simulink model "distillmpcbasic"  (Simulink 6.6)
settings: Solver=ode45  StartTime=0.0  StopTime=100.0  RelTol=1e-3
values from neighbouring files (symbols this model uses):
  alpha = 2.993    [distilldata.mat]
  F = block.DialogPrm(1).Data    [mympccontroller.m]    (also in run_lab3_5_1.m = sysd.A; run_lab3_5_2.m = sysd.A; run_lab3_5_3.m = sysd.A)
  F0 = 1    [distilldata.mat]
  G = block.DialogPrm(2).Data    [mympccontroller.m]    (also in run_lab3_5_1.m = sysd.B; run_lab3_5_2.m = sysd.B; run_lab3_5_3.m = sysd.B)
  L0 = 2    [distilldata.mat]
  M = 5    [distilldata.mat]    (also in mympccontroller.m = block.DialogPrm(3).Data; upg_10_1.m = eye(m); upg_10_2.m = eye(m))
  M0B = 10    [distilldata.mat]
  M0D = 10    [distilldata.mat]
  Mz = [1 0 0 0 0 0 0 0 0 0 0 0 ... (16 elements, 2x8)]    [distilldata.mat]    (also in run_lab3_5_3.m = [Mz, zeros(size(Mz,1),1); zeros(1,size(Mz,2)), 1])
  N = block.DialogPrm(4).Data    [mympccontroller.m]    (also in results_51.mat = 20; run_lab3_5_1.m = 20; run_lab3_5_2.m = 70; run_lab3_5_3.m = 70)
  Q1 = block.DialogPrm(5).Data    [mympccontroller.m]    (also in run_lab3_5_1.m = eye(size(Mz,1)); run_lab3_5_2.m = diag([110, 200]); run_lab3_5_3.m = diag([110, 200, q_z3]); upg_10_1.m = 10*eye(m))
  Q2 = block.DialogPrm(6).Data    [mympccontroller.m]    (also in run_lab3_5_1.m = 1e-2*eye(size(G,2)); run_lab3_5_2.m = 6e-4*eye(m); run_lab3_5_3.m = diag([1,1 1000]); upg_10_1.m = 0.1)
  Ts = block.DialogPrm(8).Data    [mympccontroller.m]    (also in results_51.mat = 1; run_lab3_5_1.m = 1; run_lab3_5_2.m = 1; run_lab3_5_3.m = 1)
  ubounds = block.DialogPrm(7).Data    [mympccontroller.m]    (also in results_51.mat = [-2.5  2.5; -2  3]; run_lab3_5_1.m = [ -V0, 5 - V0; run_lab3_5_2.m = [ -V0, 5 - V0; run_lab3_5_3.m = [ -V0, 5 - V0)
  V0 = 2.5    [distilldata.mat]
  x0 = [0.9577452092 0.883354566 0.7467709401 0.5553784995 0.3912960402 0.2223240273 0.1042469935 0.04225479085]    [distilldata.mat]    (also in run_lab3_5_1.m = xdagger; run_lab3_5_2.m = xstar(:); run_lab3_5_3.m = xstar(:))
  xF0 = 0.5    [distilldata.mat]
  xstar = [0.9577452092 0.883354566 0.7467709401 0.5553784995 0.3912960402 0.2223240273 0.1042469935 0.04225479085]    [distilldata.mat]
settings Model: Creator=maren  LastModifiedBy=maren  ExtModeAutoUpdateStatusClock=off

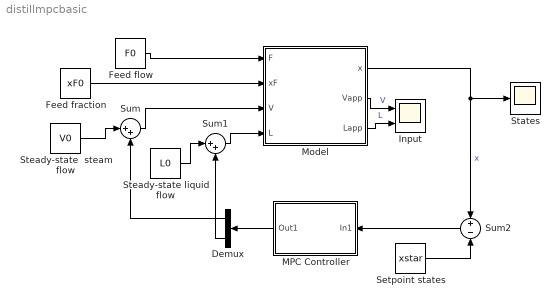
== system distillmpcbasic ==
  Demux : Demux  Orientation=left  Outputs=2
  Feed flow : Constant  Value=F0
  Feed fraction : Constant  Value=xF0
  Input : Scope  NumInputPorts=2
      settings: TimeRange=100  YMin=2.5~2  YMax=5~2.125  SaveName=U
  MPC Controller : Subsystem  Orientation=left  mask{F=F, G=G, M=Mz, N=N, Q1=Q1, Q2=Q2, ubounds=ubounds, Ts=Ts, ufname='solvempcproblem'}
      mask prompts: ubounds "Input bounds [u1min u1max;u2min u2max;...]"; ufname "Output function (Ex: 'myfun1')"
      mask Display:
      | port_label('input',1,'x')
      | port_label('output',1,'u')
  Model : Subsystem
  Setpoint states : Constant  Value=xstar
  States : Scope
      settings: TimeRange=100  YMin=0  YMax=1  SaveName=X
  Steady-state liquid flow : Constant  Value=L0
  Steady-state  steam flow : Constant  Value=V0
  Sum : Sum  Inputs=|++  SaturateOnIntegerOverflow=on
  Sum1 : Sum  Inputs=|++  SaturateOnIntegerOverflow=on
  Sum2 : Sum  Orientation=left  Inputs=+-  SaturateOnIntegerOverflow=on
  wires:
  Feed flow/1 -> Model/1(F)
  Feed fraction/1 -> Model/2(xF)
  Steady-state  steam flow/1 -> Sum/1
  Sum/1 -> Model/3(V)
  Demux/1 -> Sum/2
  Steady-state liquid flow/1 -> Sum1/1
  Demux/2 -> Sum1/2
  Sum1/1 -> Model/4(L)
  Model/1(x) -> States/1, Sum2/1  "x"
  Setpoint states/1 -> Sum2/2
  Model/2(Vapp) -> Input/1  "V"
  Model/3(Lapp) -> Input/2  "L"
  MPC Controller/1(Out1) -> Demux/1
  Sum2/1 -> MPC Controller/1(In1)

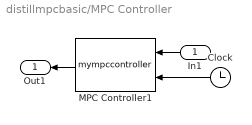
== system distillmpcbasic/MPC Controller ==
  In1 : Inport  Orientation=left
  Clock : Clock
      settings: Decimation=10
  MPC Controller1 : M-S-Function  Orientation=left  FunctionName=mympccontroller  Parameters=F,G,M,N,Q1,Q2,ubounds,Ts,ufname  mask{F=F, G=G, M=M, N=N, Q1=Q1, Q2=Q2, ubounds=ubounds, Ts=Ts, ufname=ufname}
      mask prompts: ubounds "ubounds [u1min u1max;u2min u2max;...]"; ufname "Output function (Ex: 'myfun1')"
      mask Display:
      | port_label('input',1,'x')
      | port_label('input',2,'t')
      | port_label('output',1,'u')
  Out1 : Outport  Orientation=left
  wires:
  Clock/1 -> MPC Controller1/2
  In1/1 -> MPC Controller1/1
  MPC Controller1/1 -> Out1/1

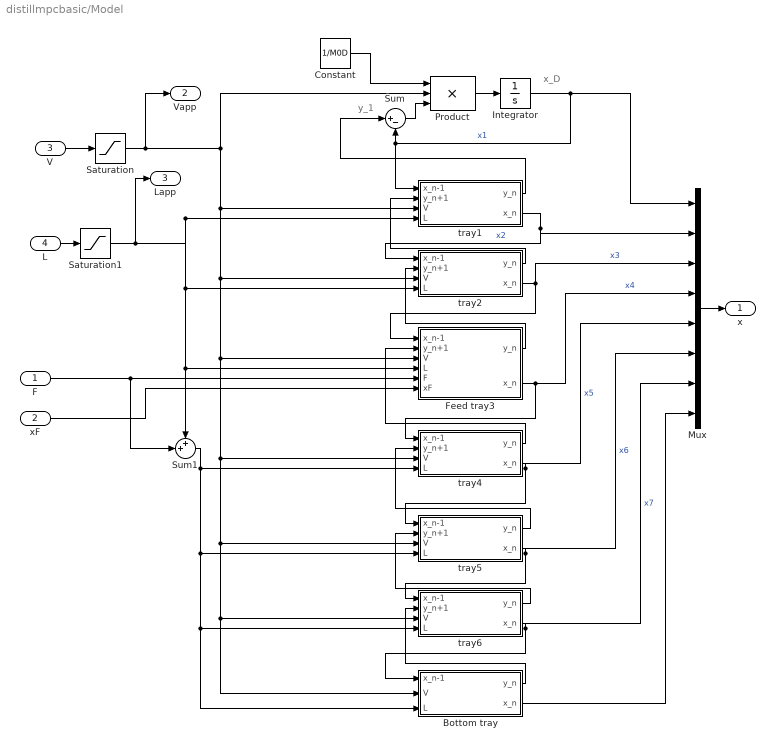
== system distillmpcbasic/Model ==
  note: y_1
  note: x_D
  F : Inport
  xF : Inport  Port=2
  V : Inport  Port=3
  L : Inport  Port=4
  Bottom tray : Subsystem
  Constant : Constant  Value=1/M0D
  Feed tray3 : Subsystem
  Integrator : Integrator  InitialCondition=x0(1)
  Mux : Mux  Inputs=8
  Product : Product  Inputs=3  SaturateOnIntegerOverflow=on
  Saturation : Saturate  UpperLimit=5  LowerLimit=0
  Saturation1 : Saturate  UpperLimit=5  LowerLimit=0
  Sum : Sum  Inputs=|+-  SaturateOnIntegerOverflow=on
  Sum1 : Sum  Inputs=++|  SaturateOnIntegerOverflow=on
  tray1 : Subsystem
  tray2 : Subsystem
  tray4 : Subsystem
  tray5 : Subsystem
  tray6 : Subsystem
  x : Outport
  Vapp : Outport  Port=2
  Lapp : Outport  Port=3
  wires:
  L/1 -> Saturation1/1
  V/1 -> Saturation/1
  Mux/1 -> x/1
  Bottom tray/2(x_n) -> Mux/8
  tray6/2(x_n) -> Mux/7, Bottom tray/1(x_n-1)  "x7"
  Bottom tray/1(y_n) -> tray6/2(y_n+1)
  Sum1/1 -> Bottom tray/3(L), tray6/4(L), tray5/4(L), tray4/4(L)
  tray5/2(x_n) -> Mux/6, tray6/1(x_n-1)  "x6"
  tray6/1(y_n) -> tray5/2(y_n+1)
  tray4/2(x_n) -> Mux/5, tray5/1(x_n-1)  "x5"
  tray5/1(y_n) -> tray4/2(y_n+1)
  Feed tray3/2(x_n) -> Mux/4, tray4/1(x_n-1)  "x4"
  tray4/1(y_n) -> Feed tray3/2(y_n+1)
  xF/1 -> Feed tray3/6(xF)
  F/1 -> Sum1/2, Feed tray3/5(F)
  tray2/2(x_n) -> Mux/3, Feed tray3/1(x_n-1)  "x3"
  Feed tray3/1(y_n) -> tray2/2(y_n+1)
  tray1/2(x_n) -> Mux/2, tray2/1(x_n-1)  "x2"
  tray2/1(y_n) -> tray1/2(y_n+1)
  tray1/1(y_n) -> Sum/1
  Saturation1/1 -> Lapp/1, Sum1/1, Feed tray3/4(L), tray2/4(L), tray1/4(L)
  Saturation/1 -> Vapp/1, Bottom tray/2(V), tray6/3(V), tray5/3(V), tray4/3(V), Feed tray3/3(V), tray2/3(V), tray1/3(V), Product/2
  Sum/1 -> Product/3
  Constant/1 -> Product/1
  Product/1 -> Integrator/1
  Integrator/1 -> Mux/1, tray1/1(x_n-1), Sum/2  "x1"

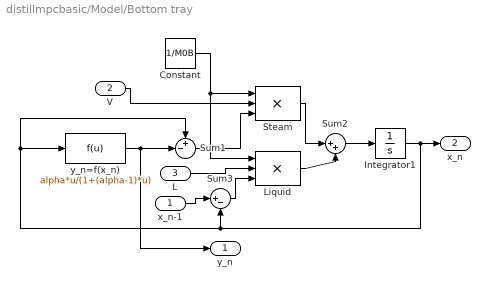
== system distillmpcbasic/Model/Bottom tray ==
  x_n-1 : Inport
  V : Inport  Port=2
  L : Inport  Port=3
  Constant : Constant  Value=1/M0B
  Integrator1 : Integrator  InitialCondition=x0(8)
  Liquid : Product  Inputs=3  SaturateOnIntegerOverflow=on
  Steam : Product  Inputs=3  SaturateOnIntegerOverflow=on
  Sum1 : Sum  Inputs=+-|  SaturateOnIntegerOverflow=on
  Sum2 : Sum  Inputs=|++  SaturateOnIntegerOverflow=on
  Sum3 : Sum  Inputs=|+-  SaturateOnIntegerOverflow=on
  y_n=f(x_n) : Fcn  Expr=alpha*u/(1+(alpha-1)*u)
  y_n : Outport
  x_n : Outport  Port=2
  wires:
  Sum1/1 -> Steam/3
  Constant/1 -> Steam/1, Liquid/1
  Integrator1/1 -> x_n/1, Sum1/1, y_n=f(x_n)/1, Sum3/2
  y_n=f(x_n)/1 -> y_n/1, Sum1/2
  V/1 -> Steam/2
  Liquid/1 -> Sum2/2
  Steam/1 -> Sum2/1
  Sum2/1 -> Integrator1/1
  L/1 -> Liquid/2
  x_n-1/1 -> Sum3/1
  Sum3/1 -> Liquid/3

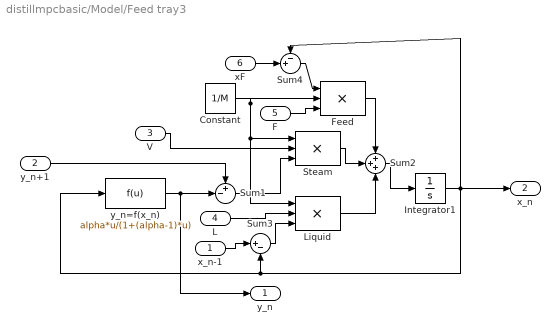
== system distillmpcbasic/Model/Feed tray3 ==
  x_n-1 : Inport
  y_n+1 : Inport  Port=2
  V : Inport  Port=3
  L : Inport  Port=4
  F : Inport  Port=5
  xF : Inport  Port=6
  Constant : Constant  Value=1/M
  Feed : Product  Inputs=3  SaturateOnIntegerOverflow=on
  Integrator1 : Integrator  InitialCondition=x0(4)
  Liquid : Product  Inputs=3  SaturateOnIntegerOverflow=on
  Steam : Product  Inputs=3  SaturateOnIntegerOverflow=on
  Sum1 : Sum  Inputs=+-|  SaturateOnIntegerOverflow=on
  Sum2 : Sum  Inputs=+++  SaturateOnIntegerOverflow=on
  Sum3 : Sum  Inputs=|+-  SaturateOnIntegerOverflow=on
  Sum4 : Sum  Inputs=-+|  SaturateOnIntegerOverflow=on
  y_n=f(x_n) : Fcn  Expr=alpha*u/(1+(alpha-1)*u)
  y_n : Outport
  x_n : Outport  Port=2
  wires:
  Feed/1 -> Sum2/1
  Sum4/1 -> Feed/1
  F/1 -> Feed/3
  xF/1 -> Sum4/2
  Steam/1 -> Sum2/2
  Liquid/1 -> Sum2/3
  Sum1/1 -> Steam/3
  Constant/1 -> Feed/2, Steam/1, Liquid/1
  Integrator1/1 -> Sum4/1, x_n/1, y_n=f(x_n)/1, Sum3/2
  y_n=f(x_n)/1 -> y_n/1, Sum1/2
  y_n+1/1 -> Sum1/1
  V/1 -> Steam/2
  Sum2/1 -> Integrator1/1
  L/1 -> Liquid/2
  x_n-1/1 -> Sum3/1
  Sum3/1 -> Liquid/3

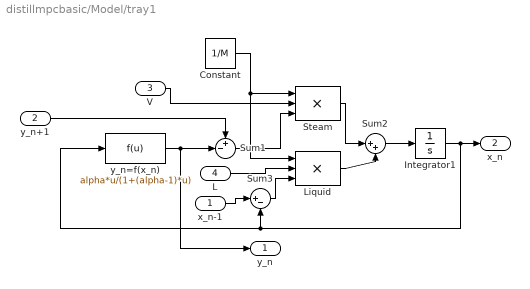
== system distillmpcbasic/Model/tray1 ==
  x_n-1 : Inport
  y_n+1 : Inport  Port=2
  V : Inport  Port=3
  L : Inport  Port=4
  Constant : Constant  Value=1/M
  Integrator1 : Integrator  InitialCondition=x0(2)
  Liquid : Product  Inputs=3  SaturateOnIntegerOverflow=on
  Steam : Product  Inputs=3  SaturateOnIntegerOverflow=on
  Sum1 : Sum  Inputs=+-|  SaturateOnIntegerOverflow=on
  Sum2 : Sum  Inputs=|++  SaturateOnIntegerOverflow=on
  Sum3 : Sum  Inputs=|+-  SaturateOnIntegerOverflow=on
  y_n=f(x_n) : Fcn  Expr=alpha*u/(1+(alpha-1)*u)
  y_n : Outport
  x_n : Outport  Port=2
  wires:
  Sum1/1 -> Steam/3
  Constant/1 -> Steam/1, Liquid/1
  Integrator1/1 -> x_n/1, y_n=f(x_n)/1, Sum3/2
  y_n=f(x_n)/1 -> y_n/1, Sum1/2
  y_n+1/1 -> Sum1/1
  V/1 -> Steam/2
  Liquid/1 -> Sum2/2
  Steam/1 -> Sum2/1
  Sum2/1 -> Integrator1/1
  L/1 -> Liquid/2
  x_n-1/1 -> Sum3/1
  Sum3/1 -> Liquid/3

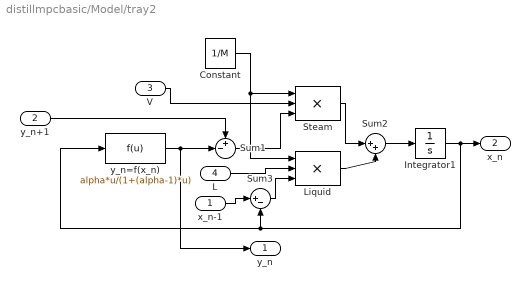
== system distillmpcbasic/Model/tray2 ==
  x_n-1 : Inport
  y_n+1 : Inport  Port=2
  V : Inport  Port=3
  L : Inport  Port=4
  Constant : Constant  Value=1/M
  Integrator1 : Integrator  InitialCondition=x0(3)
  Liquid : Product  Inputs=3  SaturateOnIntegerOverflow=on
  Steam : Product  Inputs=3  SaturateOnIntegerOverflow=on
  Sum1 : Sum  Inputs=+-|  SaturateOnIntegerOverflow=on
  Sum2 : Sum  Inputs=|++  SaturateOnIntegerOverflow=on
  Sum3 : Sum  Inputs=|+-  SaturateOnIntegerOverflow=on
  y_n=f(x_n) : Fcn  Expr=alpha*u/(1+(alpha-1)*u)
  y_n : Outport
  x_n : Outport  Port=2
  wires:
  Sum3/1 -> Liquid/3
  x_n-1/1 -> Sum3/1
  L/1 -> Liquid/2
  Sum2/1 -> Integrator1/1
  Steam/1 -> Sum2/1
  Liquid/1 -> Sum2/2
  V/1 -> Steam/2
  y_n+1/1 -> Sum1/1
  y_n=f(x_n)/1 -> Sum1/2, y_n/1
  Integrator1/1 -> Sum3/2, y_n=f(x_n)/1, x_n/1
  Constant/1 -> Liquid/1, Steam/1
  Sum1/1 -> Steam/3

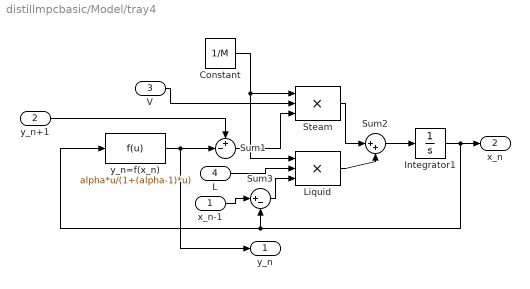
== system distillmpcbasic/Model/tray4 ==
  x_n-1 : Inport
  y_n+1 : Inport  Port=2
  V : Inport  Port=3
  L : Inport  Port=4
  Constant : Constant  Value=1/M
  Integrator1 : Integrator  InitialCondition=x0(5)
  Liquid : Product  Inputs=3  SaturateOnIntegerOverflow=on
  Steam : Product  Inputs=3  SaturateOnIntegerOverflow=on
  Sum1 : Sum  Inputs=+-|  SaturateOnIntegerOverflow=on
  Sum2 : Sum  Inputs=|++  SaturateOnIntegerOverflow=on
  Sum3 : Sum  Inputs=|+-  SaturateOnIntegerOverflow=on
  y_n=f(x_n) : Fcn  Expr=alpha*u/(1+(alpha-1)*u)
  y_n : Outport
  x_n : Outport  Port=2
  wires:
  Sum3/1 -> Liquid/3
  x_n-1/1 -> Sum3/1
  L/1 -> Liquid/2
  Sum2/1 -> Integrator1/1
  Steam/1 -> Sum2/1
  Liquid/1 -> Sum2/2
  V/1 -> Steam/2
  y_n+1/1 -> Sum1/1
  y_n=f(x_n)/1 -> Sum1/2, y_n/1
  Integrator1/1 -> Sum3/2, y_n=f(x_n)/1, x_n/1
  Constant/1 -> Liquid/1, Steam/1
  Sum1/1 -> Steam/3

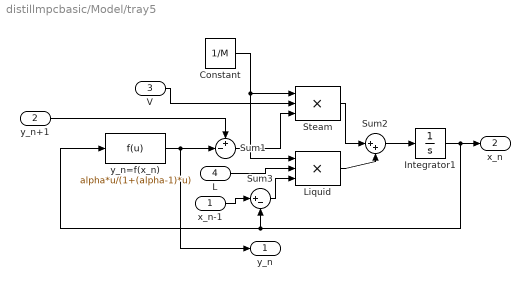
== system distillmpcbasic/Model/tray5 ==
  x_n-1 : Inport
  y_n+1 : Inport  Port=2
  V : Inport  Port=3
  L : Inport  Port=4
  Constant : Constant  Value=1/M
  Integrator1 : Integrator  InitialCondition=x0(6)
  Liquid : Product  Inputs=3  SaturateOnIntegerOverflow=on
  Steam : Product  Inputs=3  SaturateOnIntegerOverflow=on
  Sum1 : Sum  Inputs=+-|  SaturateOnIntegerOverflow=on
  Sum2 : Sum  Inputs=|++  SaturateOnIntegerOverflow=on
  Sum3 : Sum  Inputs=|+-  SaturateOnIntegerOverflow=on
  y_n=f(x_n) : Fcn  Expr=alpha*u/(1+(alpha-1)*u)
  y_n : Outport
  x_n : Outport  Port=2
  wires:
  Sum1/1 -> Steam/3
  Constant/1 -> Steam/1, Liquid/1
  Integrator1/1 -> x_n/1, y_n=f(x_n)/1, Sum3/2
  y_n=f(x_n)/1 -> y_n/1, Sum1/2
  y_n+1/1 -> Sum1/1
  V/1 -> Steam/2
  Liquid/1 -> Sum2/2
  Steam/1 -> Sum2/1
  Sum2/1 -> Integrator1/1
  L/1 -> Liquid/2
  x_n-1/1 -> Sum3/1
  Sum3/1 -> Liquid/3

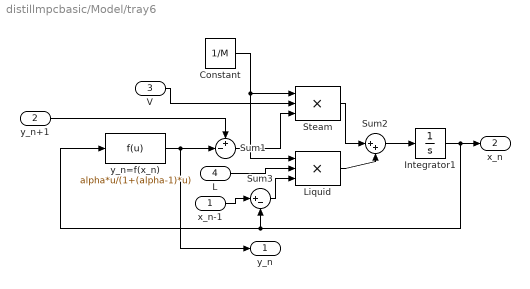
== system distillmpcbasic/Model/tray6 ==
  x_n-1 : Inport
  y_n+1 : Inport  Port=2
  V : Inport  Port=3
  L : Inport  Port=4
  Constant : Constant  Value=1/M
  Integrator1 : Integrator  InitialCondition=x0(7)
  Liquid : Product  Inputs=3  SaturateOnIntegerOverflow=on
  Steam : Product  Inputs=3  SaturateOnIntegerOverflow=on
  Sum1 : Sum  Inputs=+-|  SaturateOnIntegerOverflow=on
  Sum2 : Sum  Inputs=|++  SaturateOnIntegerOverflow=on
  Sum3 : Sum  Inputs=|+-  SaturateOnIntegerOverflow=on
  y_n=f(x_n) : Fcn  Expr=alpha*u/(1+(alpha-1)*u)
  y_n : Outport
  x_n : Outport  Port=2
  wires:
  Sum3/1 -> Liquid/3
  x_n-1/1 -> Sum3/1
  L/1 -> Liquid/2
  Sum2/1 -> Integrator1/1
  Steam/1 -> Sum2/1
  Liquid/1 -> Sum2/2
  V/1 -> Steam/2
  y_n+1/1 -> Sum1/1
  y_n=f(x_n)/1 -> Sum1/2, y_n/1
  Integrator1/1 -> Sum3/2, y_n=f(x_n)/1, x_n/1
  Constant/1 -> Liquid/1, Steam/1
  Sum1/1 -> Steam/3
